simulink model "localization_and_state_estimation"  (R2023a)
settings: Solver=ode1  StartTime=0.0  StopTime=inf  FixedStep=1/60  RelTol=1e-3  EnableMultiTasking=on
model workspace (MAT data in the model file):
  downCamStepSize : Simulink.Parameter (value not decoded)
  lidarStepSize : Simulink.Parameter (value not decoded)
  mainStepSize : Simulink.Parameter (value not decoded)
  mode : Simulink.Parameter (value not decoded)
  realSenseStepSize : Simulink.Parameter (value not decoded)
symbols that are objects in the model workspace (value not decoded): downCamStepSize, lidarStepSize, mainStepSize, mode, realSenseStepSize
undefined symbols (not defined in the file): gcbh, JPEG, Point, video_display_show
libraries: quarc_library x33, simulink x2
(part 2 of 2)

== matlab function localization_and_state_estimation/Image Processing (Line Following)/colorize ==
  data: Binary input; y output; Color input
function y = fcn(Binary, Color)

y = Color;
[ROW, COL, ~] = size(y);

y(51:100, 1:COL, 1) = ((255 - Binary)/255).*Color(51:100,:,1) + (Binary).*Color(51:100, :, 1);
y(51:100, 1:COL, 2) = ((255 - Binary)/255).*Color(51:100,:,2);
y(51:100, 1:COL, 3) = ((255 - Binary)/255).*Color(51:100,:,3);
